simulink model "problem3"  (R2020b)
settings: Solver=VariableStepAuto  StartTime=0.0  StopTime=10.0  RelTol=1e-3
settings Model: Creator=admin  LastModifiedBy=admin
settings DataIOCC: ExternalInput=[t, freq]  LoadExternalInput=on  SaveFormat=Array

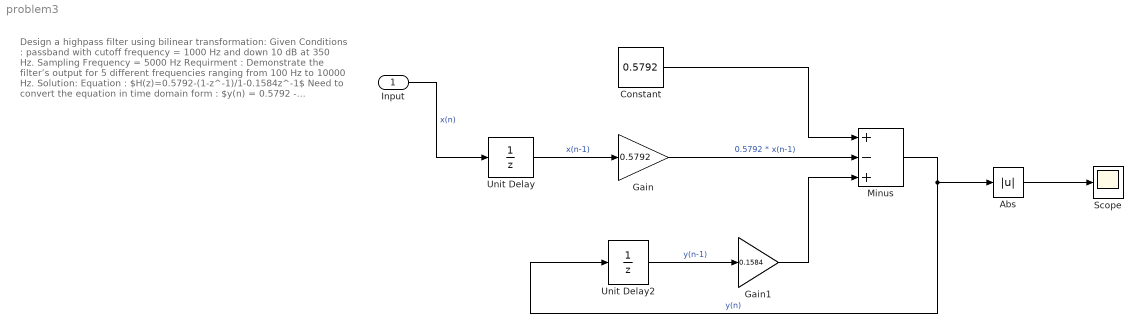
== system problem3 ==
  note: Design a highpass filter using bilinear transformation:
      |
      | Given Conditions :
      | passband with cutoff frequency = 1000 Hz
      | and down 10 dB at 350 Hz.
      | Sampling Frequency = 5000 Hz
      |
      | Requirment :
      | Demonstrate the filter’s output for 5 different frequencies ranging from 100 Hz to 10000 Hz.
      |
      | Solution:
      | Equation :
      | $H(z)=0.5792-(1-z^-1)/1-0.1584z^-1$
      |
      | Need to convert the equation in time domain form :
      |
      | $y(n) = 0.5792 - 0.5792*x(n-1) + 0.1584 * y(n-1)$
  Input : Inport
  Abs : Abs
  Constant : Constant  Value=0.5792
  Gain : Gain  Gain=0.5792
  Gain1 : Gain  Gain=0.1584
  Minus : Sum  Inputs=+-+
  Scope : Scope
  Unit Delay : UnitDelay  SampleTime=-1  HasFrameUpgradeWarning=on
  Unit Delay2 : UnitDelay  SampleTime=-1  HasFrameUpgradeWarning=on
  wires:
  Unit Delay/1 -> Gain/1  "x(n-1)"
  Input/1 -> Unit Delay/1  "x(n)"
  Gain/1 -> Minus/2  "0.5792 * x(n-1)"
  Constant/1 -> Minus/1
  Minus/1 -> Abs/1, Unit Delay2/1  "y(n)"
  Unit Delay2/1 -> Gain1/1  "y(n-1)"
  Gain1/1 -> Minus/3
  Abs/1 -> Scope/1
